simulink library "microdaq_lib"  (R2013a)
settings: Solver=ode45  SolverMode=SingleTasking  StartTime=0.0  StopTime=10.0  RelTol=1e-3
libraries: etargetslib x4
settings Model: Creator=bas  LastModifiedBy=skibool

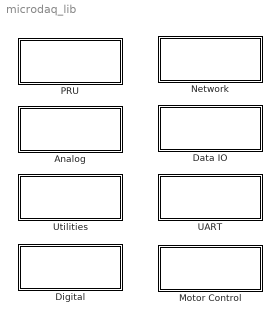
== system microdaq_lib ==
  Analog : Subsystem
  Data IO : Subsystem
  Digital : Subsystem
  Motor Control : Subsystem
  Network : Subsystem
  PRU : Subsystem
  UART : Subsystem
  Utilities : Subsystem

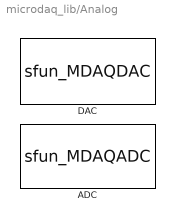
== system microdaq_lib/Analog ==
  ADC : S-Function  FunctionName=sfun_MDAQADC  Parameters=Converter, Channel, ChannelCount, Range, Polarity, Mode, SampleTime  EnableBusSupport=off  mask(ADC block){pChannel=[ 1 ], pChannelCount=ones([1 1 ]), pRange=10V | 10.24V, pPolarity=Bipolar, pMode=Single-ended, SampleTime=-1}
      mask prompts: pChannel "Channels:"; pChannelCount "ChannelCount"; pRange "Range:"; pPolarity "Polarity:"; pMode "Mode:"; SampleTime "Sample time (-1 for inherited):"
      mask help: This block reads MicroDAQ analog inputs (AI). Select ADC parameters according to your hardware setup. Block supports input ranges which differs for converter type. When 10V | 10.24V range selected depending on your ADC converter input range can be 10V or 10.24V.
      mask init:
      | Converter = 1;
      | Channel = pChannel;
      | ChannelCount = prod(size([pChannel]));
      | Polarity = pPolarity;
      | Range = pRange;
      | Mode = pMode;
      mask Help: <p>This block reads MicroDAQ analog inputs. Block supports different types of MicroDAQ analog inputs. In order to read more then one ADC channel provide array of channels to read in block 'Channels' parameter. Depending on 'Range' and 'Polarity' analog input range can be selected.</p>
      mask TypeOptions pRange: 10V | 10.24V | 5V | 5.12V | 2V | 2.56V | 1V | 1.28V | 0.64V
      mask TypeOptions pPolarity: Unipolar | Bipolar
      mask TypeOptions pMode: Single-ended | Differential
      mask Display:
      | color('blue');
      | text(0.05, 0.12, 'MicroDAQ', 'horizontalalignment', 'left');
      | color('black');
      | fprintf('\nADC\n\n\n\n');
      | color('gray');
      | 
      | 
      | fprintf('\n\nCH: %s\n\n', num2str(pChannel));
      | port_label('output',1,'Raw');
      | port_label('output',2,'Volt');
  DAC : S-Function  FunctionName=sfun_MDAQDAC  Parameters=Converter, Channel, pChannelCount, Mode, ModeTrig, TermAll, Term, SampleTime  EnableBusSupport=off  mask(DAC block){pChannel=[ 1 ], pRange=0-5V, pChannelCount=ones([1 1 ]), pTermAll=on, pTerm=0.0, SampleTime=-1}
      mask prompts: pChannel "Channels:"; pRange "Range:"; pChannelCount "ChannelCount:"; pTermAll "Terminate all DACs with voltage"; pTerm "Termination voltage:"; SampleTime "Sample time (-1 for inherited):"
      mask help:
      | This block sets MicroDAQ analog outputs (AO). DAC block allows to set terminate voltage which will be set at the end of simulation in External mode.
      |
      | User can use option Terminate all DACs with voltage to set same voltage at all DAC channels. Without selecting this option user can define different terminate voltages for DAC channel.
      |
      | Setup DAC parameters according to your hardware configuration.
      mask init:
      | Converter = 1;
      | Channel = pChannel;
      | pChannelCount = prod(size([pChannel]));
      | ModeTrig = 0;
      | TermAll = pTermAll; 
      | Term = pTerm; 
      | tmp = [0 1 4 2 3];
      | Mode = tmp(pRange);;
      mask TypeOptions pRange: 0-5V | 0-10V | ±2.5V | ±5V | ±10V
      mask Display:
      | color('blue');
      | text(0.98, 0.12, 'MicroDAQ', 'horizontalalignment', 'right');
      | color('black');
      | fprintf('\nDAC\n\n\n\n');
      | color('gray');
      | fprintf('\nCH: %s\n',num2str(pChannel));
      | port_label('input',1,'Volt');

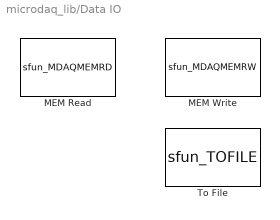
== system microdaq_lib/Data IO ==
  "MEM Read " : S-Function  FunctionName=sfun_MDAQMEMRD  Parameters=pMemAddr, pArraySize, pVectorSize, pPeriodic, SampleTime  EnableBusSupport=off  mask(Read memory block){pMemAddr=1, pArraySize=1, pVectorSize=1, Periodic=on, SampleTime=-1}
      mask prompts: pMemAddr "Start index:"; pArraySize "Size:"; pVectorSize "Vector size:"; Periodic "Circular memory buffer"; SampleTime "Sample time (-1 for inherited):"
      mask help:
      | This block reads data from MicroDAQ memory. Block with mdaq_mem_write function can be used to change Standalone model parameters.
      |
      | 'Size' parameter defines memory size used by block, e.g in order to read 1 sample of vector of size 4 user needs to set 'Size' parameter to 4 and 'Vector size' to 4.
      mask init:
      | if (Periodic)
      |     pPeriodic = 1;
      | else
      |     pPeriodic = 0;
      | end
      | 
      | pMemAddr = pMemAddr - 1;
      mask Display:
      | color('blue');
      | text(0.98, 0.13, 'MicroDAQ', 'horizontalalignment', 'right');
      | color('black');
      | fprintf('MEM Read\n\n\n');
      | color('gray');
  "MEM Write  " : S-Function  FunctionName=sfun_MDAQMEMRW  Parameters=pMemAddr, pArraySize, pVectorSize, pOverwrite, SampleTime  EnableBusSupport=off  mask(Write Memory block){pMemAddr=1, pArraySize=1, pVectorSize=1, Overwrite=on, SampleTime=-1}
      mask prompts: pMemAddr "Start index:"; pArraySize "Size:"; pVectorSize "Vector size:"; Overwrite "Circular memory buffer"; SampleTime "Sample time (-1 for inherited):"
      mask help:
      | This block writes data to MicroDAQ memory. Block with mdaq_mem_read function can be used to get data from Standalone model.
      |
      | 'Size' parameter defines memory size used by block, e.g in order to write 100 samples of vector of size 4 user needs to set 'Size' parameter to 400 and 'Vector size' to 4.
      mask init:
      | if (Overwrite)
      |     pOverwrite  = 1; 
      | else
      |     pOverwrite  = 0; 
      | end
      | pMemAddr = pMemAddr - 1;
      mask Display:
      | color('blue');
      | text(0.98, 0.13, 'MicroDAQ', 'horizontalalignment', 'right');
      | color('black');
      | fprintf('MEM Write\n\n\n');
      | color('gray');
  To File : S-Function  FunctionName=sfun_TOFILE  Parameters=pFileName, pMode, pBufSize, pVecSize, pType, SampleTime  EnableBusSupport=off  mask(To File){pName='data.txt', pType=Text, pMode=Create, pBufSize=10, pVecSize=1, SampleTime=-1}
      mask prompts: pName "File name:"; pType "Filt type:"; pMode "Mode:"; pBufSize "Vector buffer size:"; pVecSize "Vector size:"; SampleTime "Sample time (-1 for inherited):"
      mask help:
      | This block writes data to file. Files are created on user disk in 'dsp/data' directory. Files can be downloaded via web browser or mass storage interface.
      | Data can be written to file in text of binary format, data can be appended to previous content of the file or file content can be truncated. To avoid time time consuming wirte operation during every simulation step block can buffer data.
      |
      | Block parameter 'Vector buffer size' indicates how many vectors will be buffered. For example sample rate of block is 0.001sec, when user sets buffer size to 100, efective write to file will be performed every 0.1sec.
      mask init:
      | pFileName = [int8(pName),0];
      mask Help: <p>This block was generated automatically by the Legacy Code Tool. For detailed help on this tool, call<a href="matlab:legacy_code('help')"> legacy_code('help')</a>.</p>
      mask TypeOptions pType: Text | Binary
      mask TypeOptions pMode: Create | Append
      mask Display:
      | color('blue');
      | text(0.98, 0.13, 'MicroDAQ', 'horizontalalignment', 'right');
      | color('black');
      | fprintf('To File\n\n\n');
      | color('gray');
      | fprintf(pName);

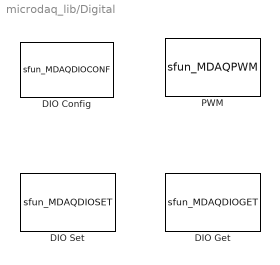
== system microdaq_lib/Digital ==
  DIO Config : S-Function  FunctionName=sfun_MDAQDIOCONF  Parameters=SParameter1, SParameter2, SParameter3, SParameter4, SParameter5, SParameter6, SParameter7, SParameter8, SParameter9, SParameter10  EnableBusSupport=off  mask(DIO Config){SParameter1=Enable, SParameter2=Enable, SParameter3=Enable, SParameter4=Enable, SParameter5=Enable, SParameter6=Enable, SParameter7=Input, SParameter8=Output, SParameter9=Output, SParameter10=Input}
      mask prompts: SParameter1 "ENC1:"; SParameter2 "ENC2:"; SParameter3 "PWM1:"; SParameter4 "PWM2:"; SParameter5 "PWM3:"; SParameter6 "UART:"; SParameter7 "DIO1...8 direction:"; SParameter8 "DIO9...16 direction:"; SParameter9 "DIO17...24 direction:"; SParameter10 "DIO25...32 direction:"
      mask help: This block configures DIO alternative functions and DIO direction.
      mask init:
      | SParameter1 = SParameter1 - 1;
      | SParameter2 = SParameter2 - 1;
      | SParameter3 = SParameter3 - 1;
      | SParameter4 = SParameter4 - 1;
      | SParameter5 = SParameter5 - 1;
      | SParameter6 = SParameter6 - 1;
      | SParameter7 = SParameter7 - 1;
      | SParameter8 = SParameter8 - 1;
      | SParameter9 = SParameter9 - 1;
      | SParameter10 = SParameter10 - 1;
      mask TypeOptions SParameter1: Disable | Enable
      mask TypeOptions SParameter2: Disable | Enable
      mask TypeOptions SParameter3: Disable | Enable
      mask TypeOptions SParameter4: Disable | Enable
      mask TypeOptions SParameter5: Disable | Enable
      mask TypeOptions SParameter6: Disable | Enable
      mask TypeOptions SParameter7: Output | Input
      mask TypeOptions SParameter8: Output | Input
      mask TypeOptions SParameter9: Output | Input
      mask TypeOptions SParameter10: Output | Input
      mask Display:
      | color('blue');
      | text(0.98, 0.13, 'MicroDAQ', 'horizontalalignment', 'right');
      | color('black');
      | fprintf('DIO Config\n\n');
  DIO Get : S-Function  FunctionName=sfun_MDAQDIOGET  Parameters=pDIOpin, SampleTime  EnableBusSupport=off  mask(DIO Get){pDIOpin=DIO1, SampleTime=-1}
      mask prompts: pDIOpin "DIO pin:"; SampleTime "Sample time (-1 for inherited):"
      mask help: This block reads MicroDAQ DIO input state.
      mask TypeOptions pDIOpin: DIO1 | DIO2 | DIO3 | DIO4 | DIO5 | DIO6 | DIO7 | DIO8 | DIO9 | DIO10 | DIO11 | DIO12 | DIO13 | DIO14 | DIO15 | DIO16 | DIO17 | DIO18 | DIO19 | DIO20 | DIO21 | DIO22 | DIO23 | DIO24 | DIO25 | DIO26 | DIO27 | DIO28 | DIO29 | DIO30 | DIO31 | DIO32
      mask Display:
      | color('blue');
      | text(0.98, 0.13, 'MicroDAQ', 'horizontalalignment', 'right');
      | color('black');
      | fprintf('DIO Get\n\n');
      | color('gray');
      | fprintf('\nDIO%d',pDIOpin);
  DIO Set : S-Function  FunctionName=sfun_MDAQDIOSET  Parameters=pDIOpin, pDIOdir, pDIOinitValue, pDIOtermValue SampleTime  EnableBusSupport=off  mask(DIO Set){pDIOpin=DIO1, pDIOdir=ones([1 1 ]), pDIOinitValue=Low, pDIOtermValue=Low, SampleTime=-1}
      mask prompts: pDIOpin "DIO pin number:"; pDIOdir "Direction:"; pDIOinitValue "DIO init value:"; pDIOtermValue "DIO term value:"; SampleTime "Sample time (-1 for inherited):"
      mask help: This block sets MicroDAQ DIO state.
      mask init:
      | pDIOdir = 0;
      mask TypeOptions pDIOpin: DIO1 | DIO2 | DIO3 | DIO4 | DIO5 | DIO6 | DIO7 | DIO8 | DIO9 | DIO10 | DIO11 | DIO12 | DIO13 | DIO14 | DIO15 | DIO16 | DIO17 | DIO18 | DIO19 | DIO20 | DIO21 | DIO22 | DIO23 | DIO24 | DIO25 | DIO26 | DIO27 | DIO28 | DIO29 | DIO30 | DIO31 | DIO32
      mask TypeOptions pDIOinitValue: High | Low
      mask TypeOptions pDIOtermValue: High | Low
      mask Display:
      | color('blue');
      | text(0.98, 0.13, 'MicroDAQ', 'horizontalalignment', 'right');
      | color('black');
      | fprintf('DIO Set\n\n');
      | color('gray');
      | fprintf('\nDIO%d',pDIOpin);
  PWM : S-Function  FunctionName=sfun_MDAQPWM  Parameters=pModule, pPeriod, pPolarity, SampleTime  EnableBusSupport=off  mask(PWM block){pModule=PWM1, pPeriod=1000, pPolarity=Active HIGH, SampleTime=-1}
      mask prompts: pModule "PWM module:"; pPeriod "Period [us]:"; pPolarity "Polarity:"; SampleTime "Sample time (-1 for inherited):"
      mask help:
      | This block sets MicroDAQ PWM outputs. Block controls one PWM module which contains A and B channels.
      | User can set PWM period in microseconds and select polarity of PWM waveform.
      | Block has two inputs A and B, when PWM block is configured to work with constant PERIOD input range is 0 - 100% .
      mask init:
      | pPolarity = pPolarity -1;
      mask TypeOptions pModule: PWM1 | PWM2 | PWM3
      mask TypeOptions pPolarity: Active HIGH | Active LOW
      mask Display:
      | color('blue');
      | text(0.98, 0.13, 'MicroDAQ', 'horizontalalignment', 'right');
      | color('black');
      | fprintf('PWM\n\n');
      | color('gray');
      | fprintf('\nPWM%d',pModule);
      | color('black');
      | port_label('input',1,'A');
      | port_label('input',2,'B');

== system microdaq_lib/Motor Control ==
  Encoder : S-Function  FunctionName=sfun_MDAQQEP  Parameters=pChannel, SampleTime  EnableBusSupport=off  mask(Encoder block){pChannel=ENC1, SampleTime=0}
      mask prompts: pChannel "Module:"; SampleTime "Sample time (-1 for inherited):"
      mask help: This block reads MicroDAQ quadrature encoder inputs (ENC).
      mask TypeOptions pChannel: ENC1 | ENC2
      mask Display:
      | color('blue');
      | text(0.05, 0.13, 'MicroDAQ', 'horizontalalignment', 'left');
      | color('black');
      | fprintf('Encoder\n\n');
      | color('gray');
      | fprintf('\nCH%d',pChannel);
      | color('black');
      | port_label('output',1,'Pos');
      | port_label('output',2,'Dir');
      | port_label('input',1,'Reset');
  PRU Encoder : S-Function  FunctionName=sfun_MDAQENC  Parameters=pPRU, SampleTime  EnableBusSupport=off  mask(PRU Encoder block){pPRU=PRU0, SampleTime=-1}
      mask prompts: pPRU "Run on:"; SampleTime "Sample time (-1 for inherited):"
      mask help:
      | This block reads quadrature encoder. Block uses quadrature encoder software implementation running on PRU core to extend MicroDAQ functionality. In order to use this block DIO25...32 needs to be configured as an input.
      |
      | Block works only with E1xxx series MicroDAQ devices!
      |
      | Channel 1 - DIO25, DIO26
      | Channel 2 - DIO27, DIO28
      | Channel 3 - DIO29, DIO30
      | Channel 4 - DIO31, DIO32
      mask init:
      | pPRU = pPRU - 1;
      mask TypeOptions pPRU: PRU0 | PRU1
      mask Display:
      | color('blue');
      | text(0.5, 0.1, 'MicroDAQ', 'horizontalalignment', 'center');
      | color('black');
      | fprintf('PRU Encoder\n\n');
      | color('gray');
      | color('black');
      | 
      | port_label('input',1,'Reset');
      | port_label('input',2,'Reset');
      | port_label('input',3,'Reset');
      | port_label('input',4,'Reset');
      | 
      | port_label('output',1,'Pos');
      | port_label('output',2,'Dir');
      | 
      | port_label('output',3,'Pos');
      | port_label('output',4,'Dir');
      | 
      | port_label('output',5,'Pos');
      | port_label('output',6,'Dir');
      | 
      | port_label('output',7,'Pos');
      | port_label('output',8,'Dir');

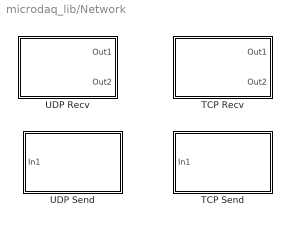
== system microdaq_lib/Network ==
  TCP Recv : Subsystem  mask(TCP/IP Recv){IPAddrStr='10.10.1.10', Port=5000, Blocking=off, Timeout=250, Datatype=double, SizePack=1, SampleTime=-1}
      mask prompts: IPAddrStr "Remote IP address:"; Port "Remote port:"; Timeout "Timeout (ms):"; Datatype "Data type:"; SizePack "Message size (in data type units):"; SampleTime "Sample time:"
      mask help: Receive TCP/IP packets from given IP port and address.
      mask init:
      | % Convert string IP Address to bytes
      | % for use in S-function
      | IPAddr = double(IPAddrStr);
      | % TCP Protocol
      | Protocol = 0;
      | % Construct data type expression for Pack block
      | %packdt = repmat({Datatype},SizePack,1);
      | packdt = {Datatype};
      | % Any better way to find data type size?
      | eval(['dummy = ',Datatype,'(0);']);
      | dummy = whos('dummy');
      | Size = SizePack*dummy.bytes;
      mask TypeOptions Datatype: double | single | uint8 | uint16 | uint32 | int8 | int16 | int32 | boolean
      mask Display:
      | color('blue');
      | text(0.98, 0.13, 'MicroDAQ', 'horizontalalignment', 'right');
      | color('black');
      | fprintf('TCP/IP Recv\n\n\n');
      | color('gray');
  TCP Send : Subsystem  mask(TCP/IP Send){IPAddrStr='10.10.1.10', Port=5000, Blocking=off, Timeout=250, Datatype=double, SizePack=1, SampleTime=-1}
      mask prompts: IPAddrStr "Remote IP address:"; Port "Remote port:"; Timeout "Timeout (ms):"; Datatype "Data type:"; SizePack "Message size (in data type units):"; SampleTime "Sample time:"
      mask help: Send TCP/IP packets to given IP port and address.
      mask init: same as microdaq_lib/Network/TCP Recv
      mask TypeOptions Datatype: double | single | uint8 | uint16 | uint32 | int8 | int16 | int32 | boolean
      mask Display:
      | color('blue');
      | text(0.98, 0.13, 'MicroDAQ', 'horizontalalignment', 'right');
      | color('black');
      | fprintf('TCP/IP Send\n\n\n');
      | color('gray');
  UDP Recv : Subsystem  mask(UDP Recv){IPAddrStr='10.10.1.10', Port=5001, Blocking=off, Timeout=250, Datatype=double, SizePack=1, SampleTime=-1}
      mask prompts: IPAddrStr "Remote IP address:"; Port "Remote port:"; Timeout "Timeout (ms):"; Datatype "Data type:"; SizePack "Message size (in data type units):"; SampleTime "Sample time:"
      mask help: Receive UDP packets from given IP port and address.
      mask init:
      | % Convert string IP Address to bytes
      | % for use in S-function
      | IPAddr = double(IPAddrStr);
      | % UDP Protocol
      | Protocol = 1;
      | % Construct data type expression for Pack block
      | %packdt = repmat({Datatype},SizePack,1);
      | packdt = {Datatype};
      | % Any better way to find data type size?
      | eval(['dummy = ',Datatype,'(0);']);
      | dummy = whos('dummy');
      | Size = SizePack*dummy.bytes;
      mask TypeOptions Datatype: double | single | uint8 | uint16 | uint32 | int8 | int16 | int32 | boolean
      mask Display:
      | color('blue');
      | text(0.98, 0.13, 'MicroDAQ', 'horizontalalignment', 'right');
      | color('black');
      | fprintf('UDP Recv\n\n\n');
      | color('gray');
  UDP Send : Subsystem  mask(UDP Send){IPAddrStr='10.10.1.10', Port=5000, Blocking=off, Timeout=250, Datatype=double, SizePack=1, SampleTime=-1}
      mask prompts: IPAddrStr "Remote IP address:"; Port "Remote port:"; Timeout "Timeout (ms):"; Datatype "Data type:"; SizePack "Message size (in data type units):"; SampleTime "Sample time:"
      mask help: Send UDP packets to given IP port and address.
      mask init: same as microdaq_lib/Network/UDP Recv
      mask TypeOptions Datatype: double | single | uint8 | uint16 | uint32 | int8 | int16 | int32 | boolean
      mask Display:
      | color('blue');
      | text(0.98, 0.13, 'MicroDAQ', 'horizontalalignment', 'right');
      | color('black');
      | fprintf('UDP Send\n\n\n');
      | color('gray');

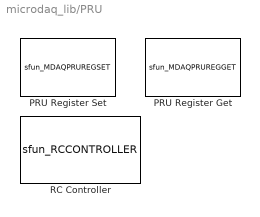
== system microdaq_lib/PRU ==
  " PRU Register Get" : S-Function  FunctionName=sfun_MDAQPRUREGGET  Parameters=pPRU, pPruRegNum, SampleTime  EnableBusSupport=off  mask(PRU Register Get){pPRU=PRU0, pPruReg=R0, SampleTime=-1}
      mask prompts: pPRU "PRU core:"; pPruReg "PRU Register"; SampleTime "Sample time (-1 for inherited):"
      mask help: This block reads MicroDAQ PRU real-time execution unit register.
      mask init:
      | pPruRegNum = pPruReg -1; 
      | pPRU = pPRU - 1;
      mask TypeOptions pPRU: PRU0 | PRU1
      mask TypeOptions pPruReg: R0 | R1 | R2 | R3 | R4 | R5 | R6 | R7 | R8 | R9 | R10 | R11 | R12 | R13 | R14 | R15
      mask Display:
      | color('blue');
      | text(0.98, 0.13, 'MicroDAQ', 'horizontalalignment', 'right');
      | color('black');
      | fprintf('PRU Reg Get\n\n');
      | color('gray');
      | fprintf('\nR%d',pPruRegNum);
  " PRU Register Set " : S-Function  FunctionName=sfun_MDAQPRUREGSET  Parameters="pPRU, pPruRegNum,  SampleTime"  EnableBusSupport=off  mask(PRU Register Set){pPRU=PRU0, pPruReg=R0, SampleTime=-1}
      mask prompts: pPRU "PRU core:"; pPruReg "PRU register:"; SampleTime "Sample time (-1 for inherited):"
      mask help: This block sets MicroDAQ PRU real-time execution unit register.
      mask init:
      | pPRU = pPRU - 1; 
      | pPruRegNum = pPruReg -1;
      mask TypeOptions pPRU: PRU0 | PRU1
      mask TypeOptions pPruReg: R0 | R1 | R2 | R3 | R4 | R5 | R6 | R7 | R8 | R9 | R10 | R11 | R12 | R13 | R14 | R15
      mask Display:
      | color('blue');
      | text(0.98, 0.13, 'MicroDAQ', 'horizontalalignment', 'right');
      | color('black');
      | fprintf('PRU Reg Set\n\n');
      | color('gray');
      | fprintf('\nR%d',pPruRegNum);
  RC Controller : S-Function  FunctionName=sfun_RCCONTROLLER  Parameters=pPRUnum, SampleTime  EnableBusSupport=off  mask(RC Controller block){pPRUnum=PRU0, SampleTime=-1}
      mask prompts: pPRUnum "Run on:"; SampleTime "Sample time (-1 for inherited):"
      mask help:
      | This block converts PWM signals from RC controller receiver to number. Block supports up to 4 PWM channels. In order to use block DIO25...DIO28 needs to be configured as an input.
      |
      | Block works only with E1xxx series MicroDAQ devices!
      |
      | Channels 1 - DIO25
      | Channels 2 - DIO26
      | Channels 3 - DIO27
      | Channels 4 - DIO28
      mask init:
      | pPRUnum = pPRUnum -1;
      mask TypeOptions pPRUnum: PRU0 | PRU1
      mask Display:
      | color('blue');
      | text(0.05, 0.13, 'MicroDAQ', 'horizontalalignment', 'left');
      | color('black');
      | fprintf('RC\nController\n');
      | 
      | color('black');
      | port_label('output',1,'Pwm');
      | port_label('output',2,'Yaw');
      | port_label('output',3,'Pitch');
      | port_label('output',4,'Throttle');

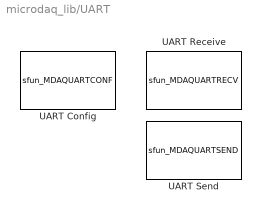
== system microdaq_lib/UART ==
  UART Config : S-Function  FunctionName=sfun_MDAQUARTCONF  Parameters=pModule, pBaudRate, pDataBits, pParity, pStopBits, pFlowControl  EnableBusSupport=off  mask(UART Config){pModule=UART0, pBaudRate=115200, pDataBits=8, pParity=None, pStopBits=1, pFlowControl=None}
      mask prompts: pModule "Module:"; pBaudRate "Baud Rate:"; pDataBits "Data bits:"; pParity "Parity:"; pStopBits "Stop bits:"; pFlowControl "Flow control:"
      mask help: This block configures MicroDAQ UART module.
      mask init:
      | pModule = pModule - 1; 
      | pDataBits = pDataBits + 4; 
      | pParity = pParity - 1;
      mask TypeOptions pModule: UART0 | UART1 | UART2
      mask TypeOptions pBaudRate: 2400 | 4800 | 9600 | 19200 | 38400 | 58600 | 115200
      mask TypeOptions pDataBits: 5 | 6 | 7 | 8
      mask TypeOptions pParity: None | Even | Odd
      mask TypeOptions pStopBits: 1 | 2
      mask TypeOptions pFlowControl: None | Hardware
      mask Display:
      | color('blue');
      | text(0.98, 0.13, 'MicroDAQ', 'horizontalalignment', 'right');
      | color('black');
      | fprintf('UART Config\n\n');
      | color('gray');
      | color('black');
  UART Receive : S-Function  FunctionName=sfun_MDAQUARTRECV  Parameters=pModule, pDataSize, pBlocking, pTimeout, pHeader, pUseHeader, SampleTime  EnableBusSupport=off  mask(UART Receive){pModule=UART0, pDataSize=16, pUseHeader=off, pHeaderStr=7161646d, pHeader=0, pBlocking=off, pTimeout=100, SampleTime=-1}
      mask prompts: pModule "Module:"; pDataSize "Data size:"; pUseHeader "Use sync data"; pHeaderStr "Sync data (32bit hex):"; pHeader "Header_p"; pBlocking "Enable blocking mode:"; pTimeout "Timeout (miliseconds):"; SampleTime "Sample time (-1 for inherited):"
      mask help:
      | This block receives data from MicroDAQ UART module. Block supports blocking and non-blocking mode. Block allows data sync with transmiter by 32bit data containing user defined value. If 'Use sync data' is enabled data output will return data stream after 32bit sync value.
      |
      | Max data size is 512 bytes.
      mask init:
      | pHeader = hex2dec(pHeaderStr);
      | pModule = pModule - 1;
      mask TypeOptions pModule: UART0 | UART1 | UART2
      mask Display:
      | color('blue');
      | text(0.05, 0.13, 'MicroDAQ', 'horizontalalignment', 'left');
      | color('black');
      | fprintf('UART\nRecv\n');
      | color('gray');
      | 
      | color('black');
      | port_label('output',1,'Data');
      | port_label('output',2,'Status');
  UART Send : S-Function  FunctionName=sfun_MDAQUARTSEND  Parameters=pModule, pDataSize, SampleTime  EnableBusSupport=off  mask(UART Send){pModule=UART0, pDataSize=16, SampleTime=1}
      mask prompts: pModule "Module:"; pDataSize "Data size:"; SampleTime "Sample time (-1 for inherited):"
      mask help: This block writes data to MicroDAQ UART module.
      mask init:
      | pModule = pModule - 1;
      mask TypeOptions pModule: UART0 | UART1 | UART2
      mask Display:
      | color('blue');
      | text(0.98, 0.13, 'MicroDAQ', 'horizontalalignment', 'right');
      | color('black');
      | fprintf('UART Send\n\n');
      | color('gray');
      | 
      | color('black');

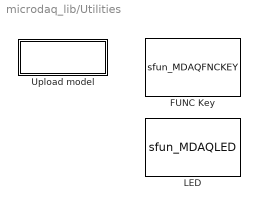
== system microdaq_lib/Utilities ==
  FUNC Key : S-Function  FunctionName=sfun_MDAQFNCKEY  Parameters=pDIOFuncKey, SampleTime  EnableBusSupport=off  mask(FUNC Key){pDIOFuncKey=F1, SampleTime=-1}
      mask prompts: pDIOFuncKey "Function key:"; SampleTime "Sample time (-1 for inherited):"
      mask help: This block allows you to read MicroDAQ function key state (F1/F2).
      mask Help: <p>This block was generated automatically by the Legacy Code Tool. For detailed help on this tool, call<a href="matlab:legacy_code('help')"> legacy_code('help')</a>.</p>
      mask TypeOptions pDIOFuncKey: F1 | F2
      mask Display:
      | color('blue');
      | text(0.98, 0.13, 'MicroDAQ', 'horizontalalignment', 'right');
      | color('black');
      | fprintf('FUNC Key\n\n');
      | color('gray');
      | fprintf('\nF%d',pDIOFuncKey);
  LED : S-Function  FunctionName=sfun_MDAQLED  Parameters=SParameter1  EnableBusSupport=off  mask(LED){SParameter1=D1}
      mask prompts: SParameter1 "Choose LED:"
      mask help:
      | This block allows you to control the built-in LEDs of MicroDAQ.
      | Setting input to 1 will switch on the selected LED.
      mask TypeOptions SParameter1: D1 | D2
      mask Display:
      | color('blue');
      | text(0.98, 0.13, 'MicroDAQ', 'horizontalalignment', 'right');
      | color('black');
      | fprintf('LED\n\n');
      | color('gray');
      | fprintf('\nD%d',SParameter1);
  Upload model : Subsystem  mask(UPLOAD block){ShowInLibBrowser=on}
      mask help:
      | This block saves DSP application on target in non-volatile memory.
      | After MicroDAQ power up DSP application will start automatically.
      | In order to upload DSP application load model on target and than double
      | click on UPLOAD block.
      |
      | DSP application will be placed on user disk in directory 'dsp'. In order to
      | turn of autostart of DSP application connect MicroDAQ with USB cable and
      | delete 'dsp-firmware.out' file in 'dsp' directory.
      settings: OpenFcn=mlink_download('', getpref('microdaq','TargetRoot'), 1)
      mask Display: disp( 'UPLOAD' )

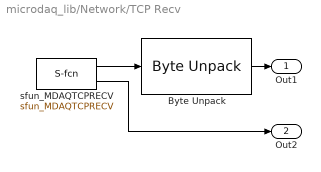
== system microdaq_lib/Network/TCP Recv ==
  Byte Unpack : etargetslib/Byte Unpack
  sfun_MDAQTCPRECV : S-Function  FunctionName=sfun_MDAQTCPRECV  Parameters=IPAddr, Port, Blocking, Timeout, Protocol, Size, SampleTime  EnableBusSupport=off
  Out1 : Outport
  Out2 : Outport  Port=2
  wires:
  sfun_MDAQTCPRECV/1 -> Byte Unpack/1
  sfun_MDAQTCPRECV/2 -> Out2/1
  Byte Unpack/1 -> Out1/1

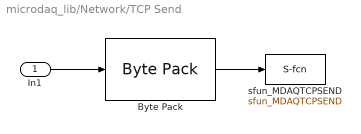
== system microdaq_lib/Network/TCP Send ==
  In1 : Inport  PortDimensions=SizePack
  Byte Pack : etargetslib/Byte Pack
  sfun_MDAQTCPSEND : S-Function  FunctionName=sfun_MDAQTCPSEND  Parameters=IPAddr, Port, Blocking, Timeout, Protocol, Size, SampleTime  EnableBusSupport=off
  wires:
  In1/1 -> Byte Pack/1
  Byte Pack/1 -> sfun_MDAQTCPSEND/1

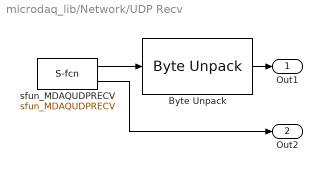
== system microdaq_lib/Network/UDP Recv ==
  Byte Unpack : etargetslib/Byte Unpack
  sfun_MDAQUDPRECV : S-Function  FunctionName=sfun_MDAQUDPRECV  Parameters=IPAddr, Port, Blocking, Timeout, Protocol, Size, SampleTime  EnableBusSupport=off
  Out1 : Outport
  Out2 : Outport  Port=2
  wires:
  Byte Unpack/1 -> Out1/1
  sfun_MDAQUDPRECV/2 -> Out2/1
  sfun_MDAQUDPRECV/1 -> Byte Unpack/1

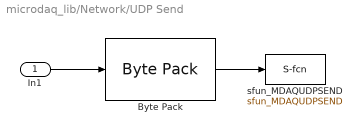
== system microdaq_lib/Network/UDP Send ==
  In1 : Inport  PortDimensions=SizePack
  Byte Pack : etargetslib/Byte Pack
  sfun_MDAQUDPSEND : S-Function  FunctionName=sfun_MDAQUDPSEND  Parameters=IPAddr, Port, Blocking, Timeout, Protocol, Size, SampleTime  EnableBusSupport=off
  wires:
  In1/1 -> Byte Pack/1
  Byte Pack/1 -> sfun_MDAQUDPSEND/1

== system microdaq_lib/Utilities/Upload model ==
  note: This block saves DSP application on target in non-volatile memory.
      | After MicroDAQ power up DSP application will start automatically.
      | In order to upload DSP application load model on target and than double
      | click on UPLOAD block.
      |
      | DSP application will be placed on user disk in directory 'dsp'. In order to
      | turn of autostart of DSP application connect MicroDAQ with USB cable and
      | delete 'dsp-firmware.out' file in 'dsp' directory.
  note: Saves DSP model on MicroDAQ
